simulink model "SimulinkControlModel"  (R2022b)
settings: Solver=VariableStepAuto  StartTime=0.0  StopTime=500  RelTol=1e-3
model workspace (MAT data in the model file):
  E = 1
  Mc = 2
  Mt = 1
  g = 9.81
  k = 1
  lamda = 0.03
undefined symbols (not defined in the file or in its folder): sigbuilder_block
libraries: slpidlib x1
settings Model: Creator=abuba  LastModifiedBy=abuba

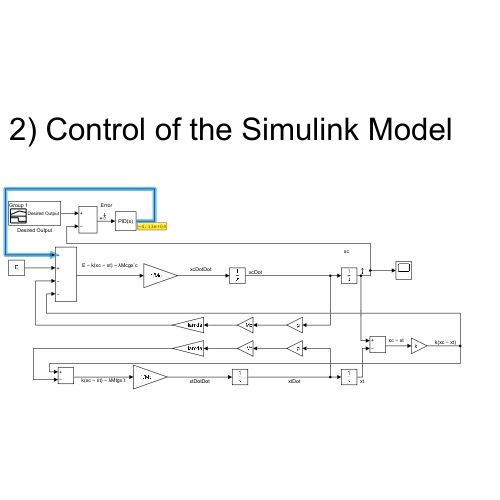
[thumbnail: Simulink's stored preview of the top-level diagram]
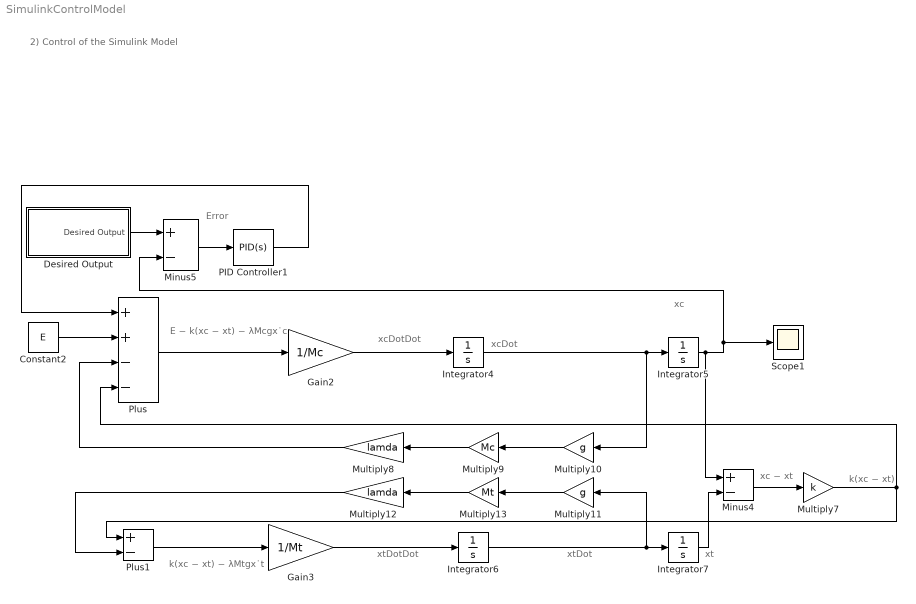
== system SimulinkControlModel ==
  note: 2) Control of the Simulink Model
  note: Error
  note: k(xc − xt) − λMtgx˙t
  note: E − k(xc − xt) − λMcgx˙c
  note: k(xc − xt)
  note: xc − xt
  note: xcDotDot
  note: xcDot
  note: xc
  note: xt
  note: xtDot
  note: xtDotDot
  Constant2 : Constant  Value=E
  Desired Output : Subsystem  Tag=STV Subsys  LoadFcn=sigbuilder_block('load',[404 199.2 550.5 362.3 ]);  StartFcn=sigbuilder_block('start');  StopFcn=sigbuilder_block('stop');  ClipboardFcn=sigbuilder_block('clipboard');  mask(Sigbuilder block){tuvar=[0:10]}
      mask help: Simulink:masks:SigbuilderBlock_MD
      mask init:
      | if ~strcmp(get_param(bdroot(gcbh),'SimulationStatus'),'stopped') tuvar = sigbuilder_block('maskInit'); end
      settings: CopyFcn=sigbuilder_block('copy');  DeleteFcn=sigbuilder_block('delete');  ModelCloseFcn=sigbuilder_block('modelClose');  PreSaveFcn=sigbuilder_block('preSave');  PauseFcn=sigbuilder_block('pause');  ContinueFcn=sigbuilder_block('continue');  NameChangeFcn=sigbuilder_block('namechange');  OpenFcn=sigbuilder_block('open',[404 199.2 550.5 362.3 ]);  CloseFcn=sigbuilder_block('close');
      mask Display: plot(0, 0, 100, 100,[2, 2, 32, 32, 2], [68, 8, 8, 68, 68],[32, 2], [38, 38], [32, 19, 2],[53, 60, 44], [32, 17, 17, 2],[16, 16, 31, 31]);txt = getActiveGroup(gcbh);text(2, 100, txt,'verticalAlignment', 'top');
  Gain2 : Gain  Gain=1/Mc
  Gain3 : Gain  Gain=1/Mt
  Integrator{4..7} (4 alike) : Integrator
  Minus4 : Sum  Inputs=+-
  Minus5 : Sum  Inputs=+-
  Multiply10 : Gain  Gain=g
  Multiply11 : Gain  Gain=g
  Multiply12 : Gain  Gain=lamda
  Multiply13 : Gain  Gain=Mt
  Multiply7 : Gain  Gain=k
  Multiply8 : Gain  Gain=lamda
  Multiply9 : Gain  Gain=Mc
  PID Controller1 : slpidlib/PID Controller  Controller=PID  Form=Parallel  TimeDomain=Continuous-time  UseExternalTs=off  SampleTime=-1  IntegratorMethod=Forward Euler  FilterMethod=Forward Euler  ControllerParametersSource=internal  P=16345.124844267  I=53209.8337437093  UseKiTs=off  D=1115.5924167861  N=63771.0241519249  UseFilter=on  TunerSelectOption=Transfer Function Based (PID Tuner App)  ZeroCross=off  InitialConditionSource=internal  InitialConditionForIntegrator=0  InitialConditionForFilter=0  DifferentiatorICPrevScaledInput=0  ExternalReset=none  TrackingMode=off  Kt=1  LimitOutput=off  SatLimitsSource=internal  UpperSaturationLimit=inf  LowerSaturationLimit=-inf  LinearizeAsGain=on  AntiWindupMode=none  Kb=1  LimitIntegrator=off  UpperIntegratorSaturationLimit=inf  LowerIntegratorSaturationLimit=-inf  POutMin=[]  POutMax=[]  IOutMin=[]  IOutMax=[]  DOutMin=[]  DOutMax=[]  NOutMin=[]  NOutMax=[]  SumOutMin=[]  SumOutMax=[]  SaturationOutMin=[]  SaturationOutMax=[]  PParamMin=[]  PParamMax=[]  IParamMin=[]  IParamMax=[]  DParamMin=[]  DParamMax=[]  NParamMin=[]  NParamMax=[]  KbParamMin=[]  KbParamMax=[]  KtParamMin=[]  KtParamMax=[]  KbOutMin=[]  KbOutMax=[]  KtOutMin=[]  KtOutMax=[]  IntegratorOutMin=[]  IntegratorOutMax=[]  FilterOutMin=[]  FilterOutMax=[]  SumI1OutMin=[]  SumI1OutMax=[]  SumI2OutMin=[]  SumI2OutMax=[]  SumI3OutMin=[]  SumI3OutMax=[]  SumI4OutMin=[]  SumI4OutMax=[]  SumDOutMin=[]  SumDOutMax=[]  DifferentiatorOutMin=[]  DifferentiatorOutMax=[]  FilterDiffOutCoefMin=[]  FilterDiffOutCoefMax=[]  ReciprocalOutMin=[]  ReciprocalOutMax=[]  SumDenOutMin=[]  SumDenOutMax=[]  SumNumOutMin=[]  SumNumOutMax=[]  DivideOutMin=[]  DivideOutMax=[]  UdiffTsProdOutMin=[]  UdiffTsProdOutMax=[]  NTsProdOutMin=[]  NTsProdOutMax=[]  UintegralTsProdOutMin=[]  UintegralTsProdOutMax=[]  UngainTsProdOutMin=[]  UngainTsProdOutMax=[]  ClampingZeroOutDataTypeStr=Inherit: Inherit via back propagation  ClampingZeroOutMin=[]  ClampingZeroOutMax=[]  FilterDenConstantOutDataTypeStr=Inherit: Inherit via back propagation  FilterDenConstantOutMin=[]  FilterDenConstantOutMax=[]  PCopyOutDataTypeStr=Inherit: Inherit via back propagation  PCopyOutMin=[]  PCopyOutMax=[]  NCopyOutDataTypeStr=Inherit: Inherit via back propagation  NCopyOutMin=[]  NCopyOutMax=[]  IntegratorContinuousStateAttributes=''  IntegratorStateMustResolveToSignalObject=off  IntegratorRTWStateStorageClass=Auto  FilterContinuousStateAttributes=''  FilterStateMustResolveToSignalObject=off  FilterRTWStateStorageClass=Auto  ParallelPVariant=InternalParameters  IdealPVariant=Disabled  IVariant=InternalParameters  DVariant=InternalParameters  IntegratorVariant=Continuous  SatVariant=Disabled  AWVariant=Passthrough  PCopyVariant=Disabled  TRVariant=Disabled  FdbkBlocksVariant=Forward  IdealPFdbkVariant=Disabled  SatFdbkVariant=Disabled  DerivativeFilterVariant=ContFilter  NVariant=InternalParameters  NCopyVariant=Disabled  FilterICVariant=InternalICsFilter  IntegratorICVariant=InternalICs  ExternalResetVariant=Disabled  TRSumVariant=Passthrough  SumFdbkVariant=Disabled  SumVariant=Sum_PID  TsampFilterVariant=InternalTs  TsampNgainVariant=Passthrough  TsampIntegralVariant=Passthrough  ExternalSaturationOutDataTypeStr=Inherit: Same as second input
  Plus : Sum  Inputs=++--
  Plus1 : Sum  Inputs=+-
  Scope1 : Scope
  wires:
  Integrator4/1 -> Integrator5/1, Multiply10/1
  Integrator5/1 -> Scope1/1, Minus5/2, Minus4/1
  Integrator6/1 -> Integrator7/1, Multiply11/1
  Gain3/1 -> Integrator6/1
  Integrator7/1 -> Minus4/2
  Minus4/1 -> Multiply7/1
  Multiply7/1 -> Plus1/1, Plus/4
  Multiply10/1 -> Multiply9/1
  Multiply9/1 -> Multiply8/1
  Multiply13/1 -> Multiply12/1
  Multiply11/1 -> Multiply13/1
  Plus/1 -> Gain2/1
  Multiply8/1 -> Plus/3
  Constant2/1 -> Plus/2
  Plus1/1 -> Gain3/1
  Multiply12/1 -> Plus1/2
  Desired Output/1(Desired Output) -> Minus5/1
  PID Controller1/1 -> Plus/1
  Minus5/1 -> PID Controller1/1
  Gain2/1 -> Integrator4/1

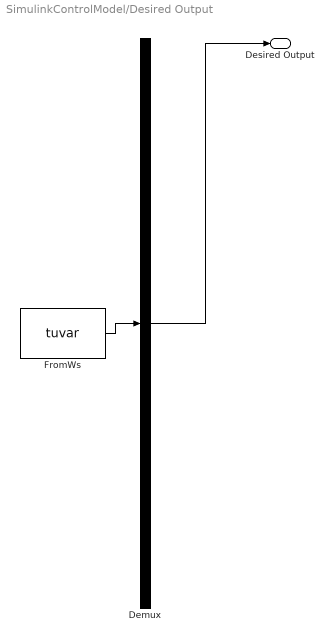
== system SimulinkControlModel/Desired Output ==
  Demux : Demux  Tag=STV Demux  Outputs=1
      settings: DisplayOption=none
  FromWs : FromWorkspace  Tag=STV FromWs  VariableName=tuvar
      SigBuilderData=|
      | common.afterFinalStr = 'Extrapolate'
      | common.sampleTime = 0
      | dataSet.timeRange = [0 500]
      | dataSet.name = 'Group 1'
      | sbobj.Groups.Name = 'Group 1'
      | sbobj.Groups.Signals.Name = 'Desired Output'
      | sbobj.Groups.Signals.XData = [0 50 50 200 200 500]
      | sbobj.Groups.Signals.YData = [0 0 1 1 0 0]
      | sbobj.Groups.TimeRange = [0 500]
  Desired Output : Outport  Tag=STV Outport
  wires:
  Demux/1 -> Desired Output/1
  FromWs/1 -> Demux/1
